simulink model "SystemModel"  (R2018b)
settings: configuration reference "FixedStepConfiguration" (kept outside this file)
settings Model: DataDictionary=DataDictionary.sldd  Creator=chris  LastModifiedBy=chris

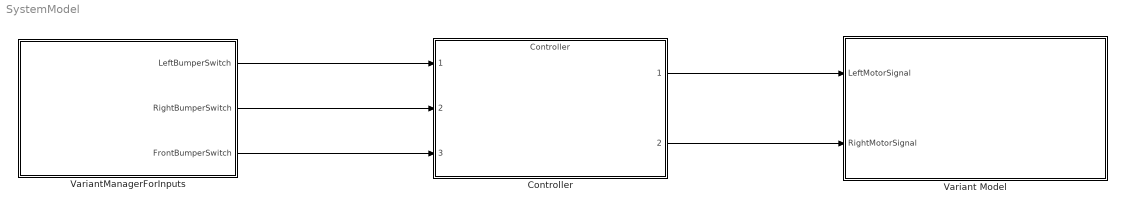
== system SystemModel ==
  Controller : ModelReference  ModelNameDialog=Controller.slx  SimulationMode=Normal  ModelReferenceVersion=1.4
  Variant Model : Subsystem  Variant=on
  VariantManagerForInputs : Subsystem  Variant=on
  wires:
  VariantManagerForInputs/1(LeftBumperSwitch) -> Controller/1
  VariantManagerForInputs/2(RightBumperSwitch) -> Controller/2
  VariantManagerForInputs/3(FrontBumperSwitch) -> Controller/3
  Controller/1 -> Variant Model/1(LeftMotorSignal)
  Controller/2 -> Variant Model/2(RightMotorSignal)

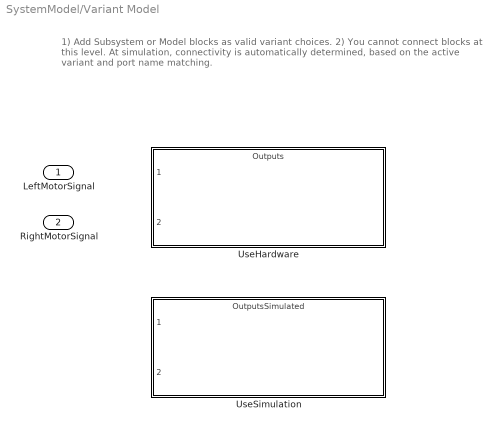
== system SystemModel/Variant Model ==
  note: 1) Add Subsystem or Model blocks as valid variant choices.
      | 2) You cannot connect blocks at this level. At simulation, connectivity is automatically
      | determined, based on the active variant and port name matching.
  LeftMotorSignal : Inport
  RightMotorSignal : Inport  Port=2
  UseHardware : ModelReference  ModelNameDialog=Outputs.slx  SimulationMode=Normal  VariantControl=UseArduino == true  ModelReferenceVersion=1.4
  UseSimulation : ModelReference  ModelNameDialog=OutputsSimulated.slx  SimulationMode=Normal  VariantControl=(default)  ModelReferenceVersion=1.2

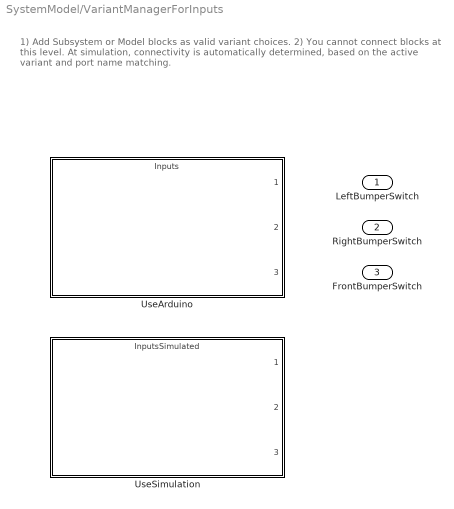
== system SystemModel/VariantManagerForInputs ==
  note: 1) Add Subsystem or Model blocks as valid variant choices.
      | 2) You cannot connect blocks at this level. At simulation, connectivity is automatically
      | determined, based on the active variant and port name matching.
  UseArduino : ModelReference  ModelNameDialog=Inputs.slx  SimulationMode=Normal  VariantControl=UseArduino == true  ModelReferenceVersion=1.2
  UseSimulation : ModelReference  ModelNameDialog=InputsSimulated.slx  SimulationMode=Normal  VariantControl=(default)  ModelReferenceVersion=1.8
  LeftBumperSwitch : Outport
  RightBumperSwitch : Outport  Port=2
  FrontBumperSwitch : Outport  Port=3
